simulink model "testfile_orb_on_Euclid"  (R2015b)
settings: Solver=VariableStepAuto  StartTime=0.0  StopTime=Inf  RelTol=1e-3
undefined symbols (not defined in the file or in its folder): motion_capture_rate, odom, realsense
libraries: genomix x4
settings Model: Creator=smishra  LastModifiedBy=smishra

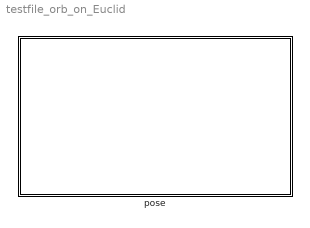
== system testfile_orb_on_Euclid ==
  pose : Subsystem

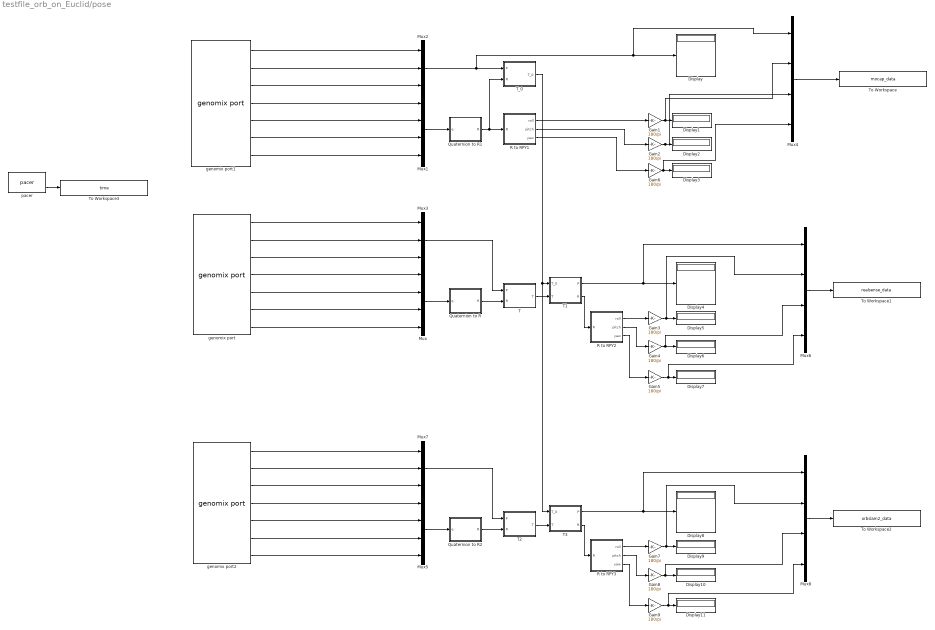
== system testfile_orb_on_Euclid/pose ==
  Display{,1..11} (12 alike) : Display
  Gain{1..9} (9 alike) : Gain  Gain=180/pi
  Mux{,1,4..6,8} (6 alike) : Mux
  Mux2 : Mux  Inputs=3
  Mux3 : Mux  Inputs=3
  Mux7 : Mux  Inputs=3
  Quaternion to R : MATLAB Function  SystemSampleTime=motion_capture_rate
  Quaternion to R1 : MATLAB Function  SystemSampleTime=motion_capture_rate
  Quaternion to R2 : MATLAB Function  SystemSampleTime=motion_capture_rate
  R to RPY1 : MATLAB Function  TreatAsAtomicUnit=on
  R to RPY2 : MATLAB Function  TreatAsAtomicUnit=on
  R to RPY3 : MATLAB Function  TreatAsAtomicUnit=on
  T : MATLAB Function  SystemSampleTime=motion_capture_rate
  T1 : MATLAB Function  SystemSampleTime=motion_capture_rate
  T2 : MATLAB Function  SystemSampleTime=motion_capture_rate
  T3 : MATLAB Function  SystemSampleTime=motion_capture_rate
  T_0 : MATLAB Function  SystemSampleTime=motion_capture_rate
  To Workspace : ToWorkspace  VariableName=mocap_data  SampleTime=-1
  To Workspace1 : ToWorkspace  VariableName=realsense_data  SampleTime=-1
  To Workspace2 : ToWorkspace  VariableName=orbslam2_data  SampleTime=-1
  To Workspace3 : ToWorkspace  VariableName=time  SampleTime=-1
  genomix port : genomix/genomix port  host=140.93.16.81:8081  component=manager  port=realsense/odom  sigtype=value  timetype=periodic  period=0.01  siglist="[{\"name\":\"pose.pose.position.x\",\"type\":\"value\",\"size\":1},{\"name\":\"pose.pose.position.y\",\"type\":\"value\",\"size\":1},{\"name\":\"pose.pose.position.z\",\"type\":\"value\",\"size\":1},{\"name\":\"pose.pose.orientation.w\",\"type\":\"value\",\"size\":1},{\"name\":\"pose.pose.orientation.x\",\"type\":\"value\",\"size\":1},{\"name\":\"pose.pose.orientation.y\",\"type\":\"value\",\"size\":1},{\"name\":\"pose.pose.orientation.z\",\"type\":\"value\",\"size\":1}]"
      settings: AttributesFormatString=manager/realsense/odom
  genomix port1 : genomix/genomix port  host=localhost  component=optitrack  port=bodies  subport=brunelleschi  sigtype=value  timetype=periodic  period=0.01  siglist="[{\"name\":\"bodies.pos.x\",\"type\":\"value\",\"size\":1},{\"name\":\"bodies.pos.y\",\"type\":\"value\",\"size\":1},{\"name\":\"bodies.pos.z\",\"type\":\"value\",\"size\":1},{\"name\":\"bodies.pos.qw\",\"type\":\"value\",\"size\":1},{\"name\":\"bodies.pos.qx\",\"type\":\"value\",\"size\":1},{\"name\":\"bodies.pos.qy\",\"type\":\"value\",\"size\":1},{\"name\":\"bodies.pos.qz\",\"type\":\"value\",\"size\":1}]"
      settings: AttributesFormatString=optitrack/bodies
  genomix port2 : genomix/genomix port  host=140.93.16.81:8081  component=ORB_SLAM2  port=pose  sigtype=value  timetype=periodic  period=0.01  siglist="[{\"name\":\"pose.position.x\",\"type\":\"value\",\"size\":1},{\"name\":\"pose.position.y\",\"type\":\"value\",\"size\":1},{\"name\":\"pose.position.z\",\"type\":\"value\",\"size\":1},{\"name\":\"pose.orientation.w\",\"type\":\"value\",\"size\":1},{\"name\":\"pose.orientation.x\",\"type\":\"value\",\"size\":1},{\"name\":\"pose.orientation.y\",\"type\":\"value\",\"size\":1},{\"name\":\"pose.orientation.z\",\"type\":\"value\",\"size\":1}]"
      settings: AttributesFormatString=ORB_SLAM2/pose
  pacer : genomix/pacer  Priority=0  catchup=off
  wires:
  Quaternion to R1/1(R) -> T_0/2(R), R to RPY1/1(R)
  genomix port1/1 -> Mux2/1
  genomix port1/2 -> Mux2/2
  genomix port1/3 -> Mux2/3
  genomix port/2 -> Mux3/2
  genomix port/3 -> Mux3/3
  Quaternion to R/1(R) -> T/2(R)
  Mux3/1 -> T/1(P)
  T/1(T) -> T1/2(T)
  R to RPY1/1(roll) -> Gain1/1
  Gain1/1 -> Mux4/2, Display1/1
  genomix port/4 -> Mux/1
  genomix port/5 -> Mux/2
  genomix port/6 -> Mux/3
  genomix port/7 -> Mux/4
  Mux/1 -> Quaternion to R/1(q)
  genomix port1/4 -> Mux1/1
  genomix port1/5 -> Mux1/2
  genomix port1/6 -> Mux1/3
  genomix port1/7 -> Mux1/4
  Mux1/1 -> Quaternion to R1/1(q)
  Gain2/1 -> Mux4/3, Display2/1
  R to RPY1/2(pitch) -> Gain2/1
  Gain6/1 -> Mux4/4, Display3/1
  R to RPY1/3(yaw) -> Gain6/1
  R to RPY2/1(roll) -> Gain3/1
  Gain3/1 -> Mux6/2, Display5/1
  R to RPY2/2(pitch) -> Gain4/1
  Gain4/1 -> Mux6/3, Display6/1
  T1/2(R) -> R to RPY2/1(R)
  R to RPY2/3(yaw) -> Gain5/1
  Gain5/1 -> Mux6/4, Display7/1
  Mux2/1 -> Mux4/1, Display/1, T_0/1(P)
  T1/1(P) -> Mux6/1, Display4/1
  Mux4/1 -> To Workspace/1
  Mux6/1 -> To Workspace1/1
  genomix port/1 -> Mux3/1
  genomix port2/2 -> Mux7/2
  genomix port2/3 -> Mux7/3
  Quaternion to R2/1(R) -> T2/2(R)
  Mux7/1 -> T2/1(P)
  T2/1(T) -> T3/2(T)
  genomix port2/4 -> Mux5/1
  genomix port2/5 -> Mux5/2
  genomix port2/6 -> Mux5/3
  genomix port2/7 -> Mux5/4
  Mux5/1 -> Quaternion to R2/1(q)
  R to RPY3/1(roll) -> Gain7/1
  Gain7/1 -> Mux8/2, Display9/1
  R to RPY3/2(pitch) -> Gain8/1
  Gain8/1 -> Mux8/3, Display10/1
  T3/2(R) -> R to RPY3/1(R)
  R to RPY3/3(yaw) -> Gain9/1
  Gain9/1 -> Mux8/4, Display11/1
  T_0/1(T_0) -> T3/1(T_0), T1/1(T_0)
  T3/1(P) -> Mux8/1, Display8/1
  Mux8/1 -> To Workspace2/1
  genomix port2/1 -> Mux7/1
  pacer/2 -> To Workspace3/1

== matlab function testfile_orb_on_Euclid/pose/Quaternion to R1 ==
  data: q input; R output
function R = fcn(q)

R=eye(3);

eta=q(1);
ex=q(2);
ey=q(3);
ez=q(4);

R=[2*(eta^2+ex^2)-1 2*(ex*ey-eta*ez) 2*(ex*ez+eta*ey);
2*(ex*ey+eta*ez) 2*(eta^2+ey^2)-1 2*(ey*ez-eta*ex);
2*(ex*ez-eta*ey) 2*(ey*ez+eta*ex) 2*(eta^2+ez^2)-1];

RCorrect=[1 0 0;0 -1 0; 0 0 -1];
% R=RCorrect*R;

== matlab function testfile_orb_on_Euclid/pose/R to RPY1 ==
  data: R input; roll output; pitch output; yaw output
function [roll,pitch,yaw] = fcn(R)

roll = atan2(R(3,2),R(3,3));
pitch = atan2(-R(3,1),sqrt(R(3,2)^2+R(3,3)^2));
yaw = atan2(R(2,1),R(1,1));

end

== matlab function testfile_orb_on_Euclid/pose/T_0 ==
  data: P input; R input; T_0 output
function T_0= fcn(P, R)

P = P(:);

persistent R0 P0

if (isempty(R0) && isempty(P0))
    R0 = R;
    P0 = P;
end

T_0 = [R0 P0; 0 0 0 1];
end

== matlab function testfile_orb_on_Euclid/pose/T ==
  data: P input; R input; T output
function T= fcn(P, R)

T = [R P; 0 0 0 1];

end

== matlab function testfile_orb_on_Euclid/pose/T1 ==
  data: P output; T_0 input; R output; T input
function [P, R] = fcn(T_0, T)

T = T_0*T;
R = T(1:3,1:3);
P = T(1:3,4);
end

== matlab function testfile_orb_on_Euclid/pose/R to RPY2 ==
  data: R input; roll output; pitch output; yaw output
function [roll,pitch,yaw] = fcn(R)

roll = atan2(R(3,2),R(3,3));
pitch = atan2(-R(3,1),sqrt(R(3,2)^2+R(3,3)^2));
yaw = atan2(R(2,1),R(1,1));

end

== matlab function testfile_orb_on_Euclid/pose/Quaternion to R2 ==
  data: q input; R output
function R = fcn(q)

R=eye(3);

eta=q(1);
ex=q(2);
ey=q(3);
ez=q(4);

R=[2*(eta^2+ex^2)-1 2*(ex*ey-eta*ez) 2*(ex*ez+eta*ey);
2*(ex*ey+eta*ez) 2*(eta^2+ey^2)-1 2*(ey*ez-eta*ex);
2*(ex*ez-eta*ey) 2*(ey*ez+eta*ex) 2*(eta^2+ez^2)-1];

RCorrect=[1 0 0;0 -1 0; 0 0 -1];
% R=RCorrect*R;

== matlab function testfile_orb_on_Euclid/pose/R to RPY3 ==
  data: R input; roll output; pitch output; yaw output
function [roll,pitch,yaw] = fcn(R)

roll = atan2(R(3,2),R(3,3));
pitch = atan2(-R(3,1),sqrt(R(3,2)^2+R(3,3)^2));
yaw = atan2(R(2,1),R(1,1));

end

== matlab function testfile_orb_on_Euclid/pose/T2 ==
  data: P input; R input; T output
function T= fcn(P, R)

T = [R P; 0 0 0 1];

end

== matlab function testfile_orb_on_Euclid/pose/T3 ==
  data: P output; T_0 input; R output; T input
function [P, R] = fcn(T_0, T)

T = T_0*T;
R = T(1:3,1:3);
P = T(1:3,4);
end

== matlab function testfile_orb_on_Euclid/pose/Quaternion to R ==
  data: q input; R output
function R = fcn(q)

R=eye(3);

eta=q(1);
ex=q(2);
ey=q(3);
ez=q(4);

R=[2*(eta^2+ex^2)-1 2*(ex*ey-eta*ez) 2*(ex*ez+eta*ey);
2*(ex*ey+eta*ez) 2*(eta^2+ey^2)-1 2*(ey*ez-eta*ex);
2*(ex*ez-eta*ey) 2*(ey*ez+eta*ex) 2*(eta^2+ez^2)-1];

RCorrect=[1 0 0;0 -1 0; 0 0 -1];
% R=RCorrect*R;
